simulink model "multicore_v0"  (R2025b)
settings: Solver=FixedStepDiscrete  StartTime=0.0  StopTime=0.1  FixedStep=0.001  RelTol=1e-3  EnableMultiTasking=on
undefined symbols (not defined in the file): task_table_data
settings Model: Creator=bianca  LastModifiedBy=ioana
settings SolverCC: PositivePriorityOrder=on  AutoInsertRateTranBlk=on
settings OptimizationCC: BlockReduction=off  DefaultParameterBehavior=Inlined  EnhancedBackFolding=on  PassReuseOutputArgsAs=Individual arguments  ZeroExternalMemoryAtStartup=off  ZeroInternalMemoryAtStartup=off  MaxStackSize=64  OptimizeBlockOrder=speed  DifferentSizesBufferReuse=on  OptimizationCustomize=off  EfficientTunableParamExpr=on
settings DebuggingCC: ParameterTunabilityLossMsg=error
settings HardwareCC: ProdBitPerPointer=32.0  ProdBitPerSizeT=32.0  ProdBitPerPtrDiffT=32.0  ProdLargestAtomicInteger=Long  ProdLargestAtomicFloat=Double  ProdWordSize=32.0  ProdLongLongMode=on  ProdHWDeviceType=ARM Compatible->ARM Cortex-A (32-bit)  HardwareBoardFeatureSet=SoCBlockset
settings ModelReferenceCC: ModelReferenceNumInstancesAllowed=Single
settings SFSimCC: MATLABDynamicMemAlloc=off
settings RTWCC: SystemTargetFile=ert.tlc  HardwareBoard=Xilinx Zynq ZC706 evaluation kit  TLCOptions="-aInlineSetEventsForThisBaseRateFcn=TLC_FALSE -aSuppressMultiTaskScheduler=TLC_FALSE  -aRateBasedStepFcn=0"  TemplateMakefile=ert_default_tmf  Toolchain=Linaro AArch32 Linux v6.3.1  Description=Embedded Coder
settings CodeAppCC: ForceParamTrailComments=on  IgnoreCustomStorageClasses=off  OperatorAnnotations=on  SimulinkDataObjDesc=on  SFDataObjDesc=on  InsertBlockDesc=on
settings ERTTargetCC: SubcomponentCodeInterfacePackaging=Nonreusable function

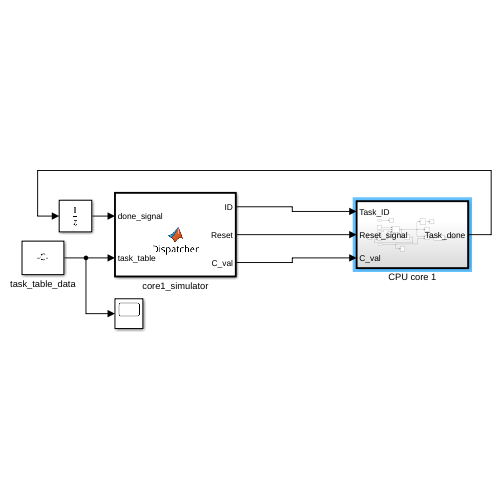
[thumbnail: Simulink's stored preview of the top-level diagram]
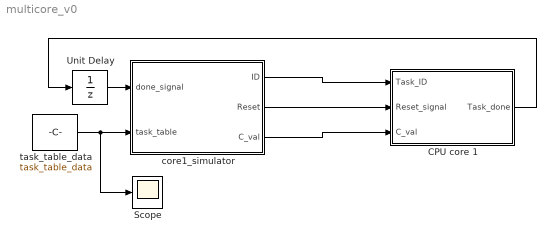
== system multicore_v0 ==
  CPU core 1 : Subsystem  TreatAsAtomicUnit=on
  Scope : Scope
      settings: ActiveDisplayYMinimum=-5.0793214612998856  ActiveDisplayYMaximum=7.391326831864939  DataLoggingSaveFormat=Array
  Unit Delay : UnitDelay  SampleTime=0.001  HasFrameUpgradeWarning=on
  core1_simulator : MATLAB Function  TreatAsAtomicUnit=on
  task_table_data : Constant  Value=task_table_data  OutDataTypeStr=double  SampleTime=0.001
  wires:
  core1_simulator/1(ID) -> CPU core 1/1(Task_ID)
  CPU core 1/1(Task_done) -> Unit Delay/1
  task_table_data/1 -> Scope/1, core1_simulator/2(task_table)
  Unit Delay/1 -> core1_simulator/1(done_signal)
  core1_simulator/3(C_val) -> CPU core 1/3(C_val)
  core1_simulator/2(Reset) -> CPU core 1/2(Reset_signal)

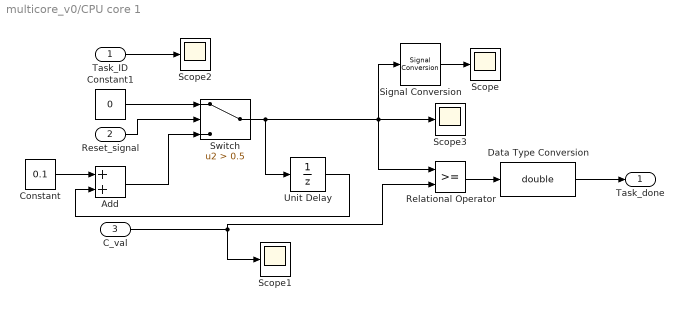
== system multicore_v0/CPU core 1 ==
  Task_ID : Inport
  Reset_signal : Inport  Port=2  PortDimensions=1
  C_val : Inport  Port=3  SampleTime=0.001
  Add : Sum
  Constant : Constant  Value=0.1  VectorParams1D=off  SampleTime=0.001
  Constant1 : Constant  Value=0
  Data Type Conversion : DataTypeConversion  OutDataTypeStr=double  SaturateOnIntegerOverflow=off  RndMeth=Floor
  Relational Operator : RelationalOperator  OutDataTypeStr=boolean  RndMeth=Simplest  InputSameDT=off
  Scope{,1..3} (4 alike) : Scope
      Scope settings: SampleTime=0.001  ActiveDisplayYMinimum=-4.7687423284474848  ActiveDisplayYMaximum=7.9290761159204077
      Scope1 settings: ActiveDisplayYMinimum=0.017801800291580072  ActiveDisplayYMaximum=1.5997230148145656
      Scope2 settings: ActiveDisplayYMinimum=0.543878907852898  ActiveDisplayYMaximum=2.6639810937715254  DataLoggingVariableName=ScopeData3
      Scope3 settings: ActiveDisplayYMinimum=-3.6924600794579923  ActiveDisplayYMaximum=7.0287315618014086  DataLoggingVariableName=ScopeData2
  Signal Conversion : SignalConversion  OverrideOpt=off
  Switch : Switch  Criteria=u2 > Threshold  Threshold=0.5  SaturateOnIntegerOverflow=off  InputSameDT=off
  Unit Delay : UnitDelay  SampleTime=-1  HasFrameUpgradeWarning=on
  Task_done : Outport
  wires:
  Switch/1 -> Relational Operator/1, Scope3/1, Signal Conversion/1, Unit Delay/1
  Relational Operator/1 -> Data Type Conversion/1
  Data Type Conversion/1 -> Task_done/1
  C_val/1 -> Relational Operator/2, Scope1/1
  Signal Conversion/1 -> Scope/1
  Constant/1 -> Add/1
  Add/1 -> Switch/3
  Reset_signal/1 -> Switch/2
  Constant1/1 -> Switch/1
  Unit Delay/1 -> Add/2
  Task_ID/1 -> Scope2/1

== matlab function multicore_v0/core1_simulator ==
  data: done_signal input size=1; ID output; task_table input; Reset output size=1; C_val output size=1
function [ID, Reset, C_val] = Dispatcher(done_signal, task_table)

    ID = 1.0;
    C_val = 0.0;
    Reset = 0.0;

    persistent current_idx;
    persistent last_done_state;

    if isempty(current_idx)
        current_idx = 1;
        last_done_state = 0;
    end

    % read inputs
    current_done = double(any(done_signal > 0.5));

    % detects whether a task is finished or not
    task_just_finished = (current_done == 1) && (last_done_state == 0);

    if task_just_finished
        current_idx = current_idx + 1;
        Reset = 1.0;
    else
        Reset = 0.0;
    end
   
    num_tasks = size(task_table, 1);
    if current_idx > num_tasks
        current_idx = 1;
    end

    last_done_state = current_done;
    
    ID = double(current_idx);

    ID = double(current_idx);
    C_val = double(task_table(current_idx, 1));
end
